simulink model "DeepWaySILForSLX_Trailer_2021a_SteerAngle"  (R2021a)
settings: Solver=FixedStepDiscrete  StartTime=0.0  StopTime=inf  FixedStep=0.001  RelTol=1e-3
InitFcn:
  | TargetIP='10.50.192.52';
libraries: simulink x14, slrealtimeutilitieslib x9, dspnetwork x4, aerolibanimutils x1
(part 2 of 2)

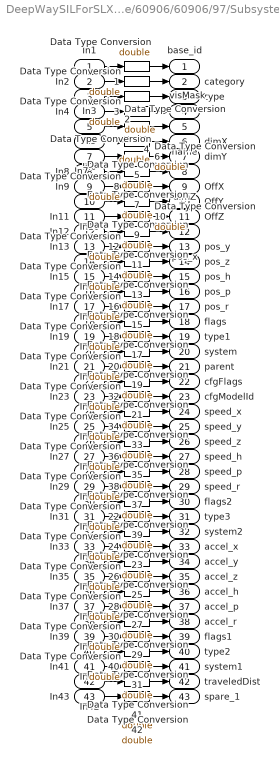
== system DeepWaySILForSLX_Trailer_2021a_SteerAngle/60906/60906/97/Subsystem1 ==
  In1 : Inport  Description=Modified By caowancang at 2021-11-19 16:04:52.
  In2 : Inport  Description=Modified By caowancang at 2021-11-19 16:04:52.  Port=2
  In3 : Inport  Description=Modified By caowancang at 2021-11-19 16:04:52.  Port=3
  In4 : Inport  Description=Modified By caowancang at 2021-11-19 16:04:52.  Port=4
  In5 : Inport  Description=Modified By caowancang at 2021-11-19 16:04:52.  Port=5
  In6 : Inport  Description=Modified By caowancang at 2021-11-19 16:04:52.  Port=6
  In7 : Inport  Description=Modified By caowancang at 2021-11-19 16:04:52.  Port=7
  In8 : Inport  Description=Modified By caowancang at 2021-11-19 16:04:52.  Port=8
  In9 : Inport  Description=Modified By caowancang at 2021-11-19 16:04:52.  Port=9
  In10 : Inport  Description=Modified By caowancang at 2021-11-19 16:04:52.  Port=10
  In11 : Inport  Description=Modified By caowancang at 2021-11-19 16:04:52.  Port=11
  In12 : Inport  Description=Modified By caowancang at 2021-11-19 16:04:52.  Port=12
  In13 : Inport  Description=Modified By caowancang at 2021-11-19 16:04:52.  Port=13
  In14 : Inport  Description=Modified By caowancang at 2021-11-19 16:04:52.  Port=14
  In15 : Inport  Description=Modified By caowancang at 2021-11-19 16:04:52.  Port=15
  In16 : Inport  Description=Modified By caowancang at 2021-11-19 16:04:52.  Port=16
  In17 : Inport  Description=Modified By caowancang at 2021-11-19 16:04:52.  Port=17
  In18 : Inport  Description=Modified By caowancang at 2021-11-19 16:04:52.  Port=18
  In19 : Inport  Description=Modified By caowancang at 2021-11-19 16:04:52.  Port=19
  In20 : Inport  Description=Modified By caowancang at 2021-11-19 16:04:52.  Port=20
  In21 : Inport  Description=Modified By caowancang at 2021-11-19 16:04:52.  Port=21
  In22 : Inport  Description=Modified By caowancang at 2021-11-19 16:04:52.  Port=22
  In23 : Inport  Description=Modified By caowancang at 2021-11-19 16:04:52.  Port=23
  In24 : Inport  Description=Modified By caowancang at 2021-11-19 16:04:52.  Port=24
  In25 : Inport  Description=Modified By caowancang at 2021-11-19 16:04:52.  Port=25
  In26 : Inport  Description=Modified By caowancang at 2021-11-19 16:04:52.  Port=26
  In27 : Inport  Description=Modified By caowancang at 2021-11-19 16:04:52.  Port=27
  In28 : Inport  Description=Modified By caowancang at 2021-11-19 16:04:52.  Port=28
  In29 : Inport  Description=Modified By caowancang at 2021-11-19 16:04:52.  Port=29
  In30 : Inport  Description=Modified By caowancang at 2021-11-19 16:04:52.  Port=30
  In31 : Inport  Description=Modified By caowancang at 2021-11-19 16:04:52.  Port=31
  In32 : Inport  Description=Modified By caowancang at 2021-11-19 16:04:52.  Port=32
  In33 : Inport  Description=Modified By caowancang at 2021-11-19 16:04:52.  Port=33
  In34 : Inport  Description=Modified By caowancang at 2021-11-19 16:04:52.  Port=34
  In35 : Inport  Description=Modified By caowancang at 2021-11-19 16:04:52.  Port=35
  In36 : Inport  Description=Modified By caowancang at 2021-11-19 16:04:52.  Port=36
  In37 : Inport  Description=Modified By caowancang at 2021-11-19 16:04:52.  Port=37
  In38 : Inport  Description=Modified By caowancang at 2021-11-19 16:04:52.  Port=38
  In39 : Inport  Description=Modified By caowancang at 2021-11-19 16:04:52.  Port=39
  In40 : Inport  Description=Modified By caowancang at 2021-11-19 16:04:52.  Port=40
  In41 : Inport  Description=Modified By caowancang at 2021-11-19 16:04:52.  Port=41
  In42 : Inport  Description=Modified By caowancang at 2021-11-19 16:04:52.  Port=42
  In43 : Inport  Description=Modified By caowancang at 2021-11-19 16:04:52.  Port=43
  Data Type Conversion{,1..42} (43 alike) : DataTypeConversion  OutDataTypeStr=double
  base_id : Outport  Description=Modified By caowancang at 2021-11-19 16:04:52.
  category : Outport  Description=Modified By caowancang at 2021-11-19 16:04:52.  Port=2
  type : Outport  Description=Modified By caowancang at 2021-11-19 16:04:52.  Port=3
  visMask : Outport  Description=Modified By caowancang at 2021-11-19 16:04:52.  Port=4
  name : Outport  Description=Modified By caowancang at 2021-11-19 16:04:52.  Port=5
  dimX : Outport  Description=Modified By caowancang at 2021-11-19 16:04:52.  Port=6
  dimY : Outport  Description=Modified By caowancang at 2021-11-19 16:04:52.  Port=7
  dimZ : Outport  Description=Modified By caowancang at 2021-11-19 16:04:52.  Port=8
  OffX : Outport  Description=Modified By caowancang at 2021-11-19 16:04:52.  Port=9
  OffY : Outport  Description=Modified By caowancang at 2021-11-19 16:04:52.  Port=10
  OffZ : Outport  Description=Modified By caowancang at 2021-11-19 16:04:52.  Port=11
  pos_x : Outport  Description=Modified By caowancang at 2021-11-19 16:04:52.  Port=12
  pos_y : Outport  Description=Modified By caowancang at 2021-11-19 16:04:52.  Port=13
  pos_z : Outport  Description=Modified By caowancang at 2021-11-19 16:04:52.  Port=14
  pos_h : Outport  Description=Modified By caowancang at 2021-11-19 16:04:52.  Port=15
  pos_p : Outport  Description=Modified By caowancang at 2021-11-19 16:04:52.  Port=16
  pos_r : Outport  Description=Modified By caowancang at 2021-11-19 16:04:52.  Port=17
  flags : Outport  Description=Modified By caowancang at 2021-11-19 16:04:52.  Port=18
  type1 : Outport  Description=Modified By caowancang at 2021-11-19 16:04:52.  Port=19
  system : Outport  Description=Modified By caowancang at 2021-11-19 16:04:52.  Port=20
  parent : Outport  Description=Modified By caowancang at 2021-11-19 16:04:52.  Port=21
  cfgFlags : Outport  Description=Modified By caowancang at 2021-11-19 16:04:52.  Port=22
  cfgModelId : Outport  Description=Modified By caowancang at 2021-11-19 16:04:52.  Port=23
  speed_x : Outport  Description=Modified By caowancang at 2021-11-19 16:04:52.  Port=24
  speed_y : Outport  Description=Modified By caowancang at 2021-11-19 16:04:52.  Port=25
  speed_z : Outport  Description=Modified By caowancang at 2021-11-19 16:04:52.  Port=26
  speed_h : Outport  Description=Modified By caowancang at 2021-11-19 16:04:52.  Port=27
  speed_p : Outport  Description=Modified By caowancang at 2021-11-19 16:04:52.  Port=28
  speed_r : Outport  Description=Modified By caowancang at 2021-11-19 16:04:52.  Port=29
  flags2 : Outport  Description=Modified By caowancang at 2021-11-19 16:04:52.  Port=30
  type3 : Outport  Description=Modified By caowancang at 2021-11-19 16:04:52.  Port=31
  system2 : Outport  Description=Modified By caowancang at 2021-11-19 16:04:52.  Port=32
  accel_x : Outport  Description=Modified By caowancang at 2021-11-19 16:04:52.  Port=33
  accel_y : Outport  Description=Modified By caowancang at 2021-11-19 16:04:52.  Port=34
  accel_z : Outport  Description=Modified By caowancang at 2021-11-19 16:04:52.  Port=35
  accel_h : Outport  Description=Modified By caowancang at 2021-11-19 16:04:52.  Port=36
  accel_p : Outport  Description=Modified By caowancang at 2021-11-19 16:04:52.  Port=37
  accel_r : Outport  Description=Modified By caowancang at 2021-11-19 16:04:52.  Port=38
  flags1 : Outport  Description=Modified By caowancang at 2021-11-19 16:04:52.  Port=39
  type2 : Outport  Description=Modified By caowancang at 2021-11-19 16:04:52.  Port=40
  system1 : Outport  Description=Modified By caowancang at 2021-11-19 16:04:52.  Port=41
  traveledDist : Outport  Description=Modified By caowancang at 2021-11-19 16:04:52.  Port=42
  spare_1 : Outport  Description=Modified By caowancang at 2021-11-19 16:04:52.  Port=43
  wires:
  In4/1 -> Data Type Conversion3/1
  Data Type Conversion3/1 -> visMask/1
  Data Type Conversion2/1 -> type/1
  In3/1 -> Data Type Conversion2/1
  In2/1 -> Data Type Conversion1/1
  Data Type Conversion1/1 -> category/1
  Data Type Conversion/1 -> base_id/1
  In1/1 -> Data Type Conversion/1
  Data Type Conversion4/1 -> name/1
  In5/1 -> Data Type Conversion4/1
  In10/1 -> Data Type Conversion9/1
  Data Type Conversion9/1 -> OffY/1
  In6/1 -> Data Type Conversion5/1
  Data Type Conversion5/1 -> dimX/1
  Data Type Conversion6/1 -> dimY/1
  In7/1 -> Data Type Conversion6/1
  In8/1 -> Data Type Conversion7/1
  Data Type Conversion7/1 -> dimZ/1
  Data Type Conversion8/1 -> OffX/1
  In9/1 -> Data Type Conversion8/1
  In19/1 -> Data Type Conversion18/1
  Data Type Conversion18/1 -> type1/1
  Data Type Conversion17/1 -> flags/1
  In18/1 -> Data Type Conversion17/1
  In17/1 -> Data Type Conversion16/1
  Data Type Conversion16/1 -> pos_r/1
  Data Type Conversion15/1 -> pos_p/1
  In16/1 -> Data Type Conversion15/1
  Data Type Conversion19/1 -> system/1
  In20/1 -> Data Type Conversion19/1
  In15/1 -> Data Type Conversion14/1
  Data Type Conversion14/1 -> pos_h/1
  In11/1 -> Data Type Conversion10/1
  Data Type Conversion10/1 -> OffZ/1
  Data Type Conversion11/1 -> pos_x/1
  In12/1 -> Data Type Conversion11/1
  In13/1 -> Data Type Conversion12/1
  Data Type Conversion12/1 -> pos_y/1
  Data Type Conversion13/1 -> pos_z/1
  In14/1 -> Data Type Conversion13/1
  In34/1 -> Data Type Conversion25/1
  Data Type Conversion25/1 -> accel_y/1
  Data Type Conversion24/1 -> accel_x/1
  In33/1 -> Data Type Conversion24/1
  In32/1 -> Data Type Conversion23/1
  Data Type Conversion23/1 -> system2/1
  Data Type Conversion22/1 -> type3/1
  In31/1 -> Data Type Conversion22/1
  Data Type Conversion26/1 -> accel_z/1
  In35/1 -> Data Type Conversion26/1
  In40/1 -> Data Type Conversion31/1
  Data Type Conversion31/1 -> type2/1
  In36/1 -> Data Type Conversion27/1
  Data Type Conversion27/1 -> accel_h/1
  Data Type Conversion28/1 -> accel_p/1
  In37/1 -> Data Type Conversion28/1
  In38/1 -> Data Type Conversion29/1
  Data Type Conversion29/1 -> accel_r/1
  Data Type Conversion30/1 -> flags1/1
  In39/1 -> Data Type Conversion30/1
  In29/1 -> Data Type Conversion38/1
  Data Type Conversion38/1 -> speed_r/1
  Data Type Conversion37/1 -> speed_p/1
  In28/1 -> Data Type Conversion37/1
  In27/1 -> Data Type Conversion36/1
  Data Type Conversion36/1 -> speed_h/1
  Data Type Conversion35/1 -> speed_z/1
  In26/1 -> Data Type Conversion35/1
  Data Type Conversion39/1 -> flags2/1
  In30/1 -> Data Type Conversion39/1
  In25/1 -> Data Type Conversion34/1
  Data Type Conversion34/1 -> speed_y/1
  In21/1 -> Data Type Conversion20/1
  Data Type Conversion20/1 -> parent/1
  Data Type Conversion21/1 -> cfgFlags/1
  In22/1 -> Data Type Conversion21/1
  In23/1 -> Data Type Conversion32/1
  Data Type Conversion32/1 -> cfgModelId/1
  Data Type Conversion33/1 -> speed_x/1
  In24/1 -> Data Type Conversion33/1
  In42/1 -> Data Type Conversion41/1
  Data Type Conversion41/1 -> traveledDist/1
  Data Type Conversion40/1 -> system1/1
  In41/1 -> Data Type Conversion40/1
  Data Type Conversion42/1 -> spare_1/1
  In43/1 -> Data Type Conversion42/1

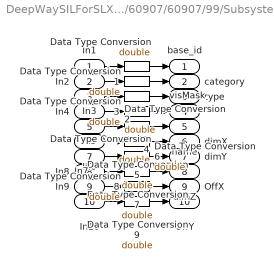
== system DeepWaySILForSLX_Trailer_2021a_SteerAngle/60907/60907/99/Subsystem1 ==
  In1 : Inport  Description=Modified By caowancang at 2021-11-19 16:04:52.
  In2 : Inport  Description=Modified By caowancang at 2021-11-19 16:04:52.  Port=2
  In3 : Inport  Description=Modified By caowancang at 2021-11-19 16:04:52.  Port=3
  In4 : Inport  Description=Modified By caowancang at 2021-11-19 16:04:52.  Port=4
  In5 : Inport  Description=Modified By caowancang at 2021-11-19 16:04:52.  Port=5
  In6 : Inport  Description=Modified By caowancang at 2021-11-19 16:04:52.  Port=6
  In7 : Inport  Description=Modified By caowancang at 2021-11-19 16:04:52.  Port=7
  In8 : Inport  Description=Modified By caowancang at 2021-11-19 16:04:52.  Port=8
  In9 : Inport  Description=Modified By caowancang at 2021-11-19 16:04:52.  Port=9
  In10 : Inport  Description=Modified By caowancang at 2021-11-19 16:04:52.  Port=10
  Data Type Conversion{,1..9} (10 alike) : DataTypeConversion  OutDataTypeStr=double
  base_id : Outport  Description=Modified By caowancang at 2021-11-19 16:04:52.
  category : Outport  Description=Modified By caowancang at 2021-11-19 16:04:52.  Port=2
  type : Outport  Description=Modified By caowancang at 2021-11-19 16:04:52.  Port=3
  visMask : Outport  Description=Modified By caowancang at 2021-11-19 16:04:52.  Port=4
  name : Outport  Description=Modified By caowancang at 2021-11-19 16:04:52.  Port=5
  dimX : Outport  Description=Modified By caowancang at 2021-11-19 16:04:52.  Port=6
  dimY : Outport  Description=Modified By caowancang at 2021-11-19 16:04:52.  Port=7
  dimZ : Outport  Description=Modified By caowancang at 2021-11-19 16:04:52.  Port=8
  OffX : Outport  Description=Modified By caowancang at 2021-11-19 16:04:52.  Port=9
  OffY : Outport  Description=Modified By caowancang at 2021-11-19 16:04:52.  Port=10
  wires:
  In9/1 -> Data Type Conversion8/1
  Data Type Conversion8/1 -> OffX/1
  Data Type Conversion7/1 -> dimZ/1
  In8/1 -> Data Type Conversion7/1
  In7/1 -> Data Type Conversion6/1
  Data Type Conversion6/1 -> dimY/1
  Data Type Conversion5/1 -> dimX/1
  In6/1 -> Data Type Conversion5/1
  Data Type Conversion9/1 -> OffY/1
  In10/1 -> Data Type Conversion9/1
  In5/1 -> Data Type Conversion4/1
  Data Type Conversion4/1 -> name/1
  In1/1 -> Data Type Conversion/1
  Data Type Conversion/1 -> base_id/1
  Data Type Conversion1/1 -> category/1
  In2/1 -> Data Type Conversion1/1
  In3/1 -> Data Type Conversion2/1
  Data Type Conversion2/1 -> type/1
  Data Type Conversion3/1 -> visMask/1
  In4/1 -> Data Type Conversion3/1
